simulink model "BallBalancingwoFb"  (R2025a)
settings: Solver=VariableStepAuto  StartTime=0.0  StopTime=10.0  RelTol=1e-3
values from neighbouring files (symbols this model uses):
  Kb = 0.028    [Lab3_BallBalancing.m]
  Km = 1    [Lab3_BallBalancing.m]
  T0 = 0.057    [Lab3_BallBalancing.m]
  z1 = timeseries(z1_signal, dt2)    [Lab3_BallBalancing.m]
  z2 = timeseries(z2_signal, dt2)    [Lab3_BallBalancing.m]
  z3 = timeseries(z3_signal, dt2)    [Lab3_BallBalancing.m]
  zeta = 0.59    [Lab3_BallBalancing.m]
settings Model: Creator=Admin  LastModifiedBy=Admin

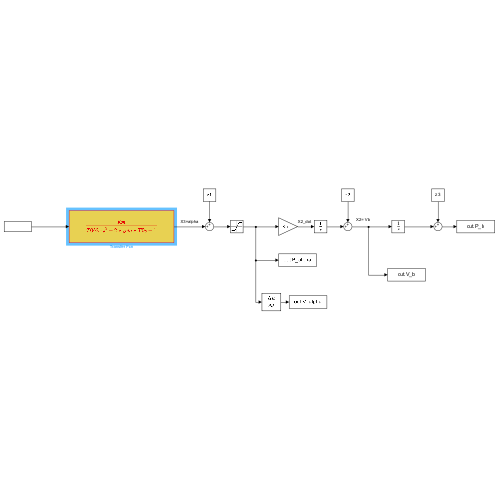
[thumbnail: Simulink's stored preview of the top-level diagram]
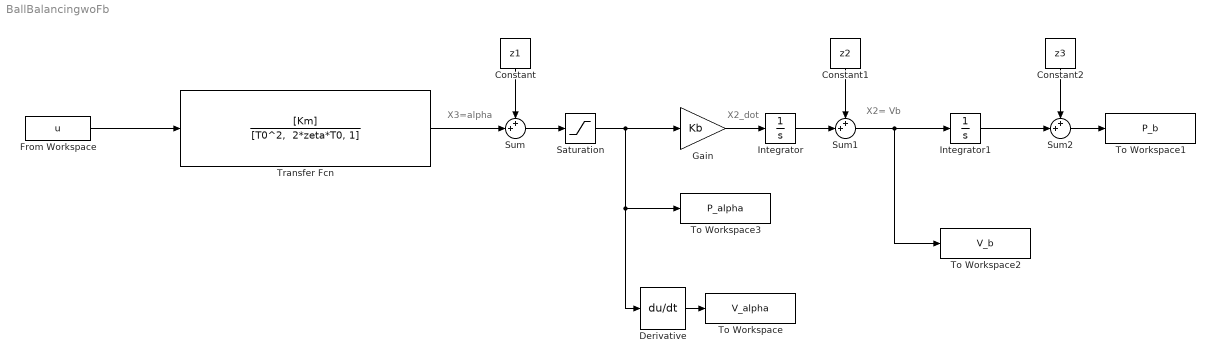
== system BallBalancingwoFb ==
  note: X3=alpha
  note: X2_dot
  note: X2= Vb
  Constant : Constant  Value=z1
  Constant1 : Constant  Value=z2
  Constant2 : Constant  Value=z3
  Derivative : Derivative
  From Workspace : FromWorkspace  VariableName=u
  Gain : Gain  Gain=Kb
  Integrator : Integrator
  Integrator1 : Integrator
  Saturation : Saturate  UpperLimit=45  LowerLimit=-45
  Sum : Sum  Inputs=++|
  Sum1 : Sum  Inputs=++|
  Sum2 : Sum  Inputs=++|
  To Workspace : ToWorkspace  VariableName=V_alpha  SaveFormat=Timeseries  SampleTime=-1
  To Workspace1 : ToWorkspace  VariableName=P_b  SaveFormat=Timeseries  SampleTime=-1
  To Workspace2 : ToWorkspace  VariableName=V_b  SaveFormat=Timeseries  SampleTime=-1
  To Workspace3 : ToWorkspace  VariableName=P_alpha  SaveFormat=Timeseries  SampleTime=-1
  Transfer Fcn : TransferFcn  Numerator=[Km]  Denominator="[T0^2,  2*zeta*T0, 1]"
  wires:
  Gain/1 -> Integrator/1
  From Workspace/1 -> Transfer Fcn/1
  Saturation/1 -> To Workspace3/1, Derivative/1, Gain/1
  Derivative/1 -> To Workspace/1
  Integrator1/1 -> Sum2/2
  Sum2/1 -> To Workspace1/1
  Integrator/1 -> Sum1/2
  Sum1/1 -> To Workspace2/1, Integrator1/1
  Constant/1 -> Sum/1
  Sum/1 -> Saturation/1
  Transfer Fcn/1 -> Sum/2
  Constant1/1 -> Sum1/1
  Constant2/1 -> Sum2/1
